simulink library "tqr"  (R2021b)
settings: Solver=VariableStepAuto  StartTime=0.0  StopTime=10.0  RelTol=1e-3
undefined symbols (not defined in the file): ATQR_AltRDCActiveFEDUInc_X_pct, ATQR_AltRDCActiveFEDUInc_Y_enum, ATQR_AltRDCActiveFEDUTs_X_pct, ATQR_AltRDCActiveFEDUTs_Y_enum, ATQR_AltRDCActiveREDUInc_X_pct, ATQR_AltRDCActiveREDUInc_Y_enum, ATQR_AltRDCActiveREDUTs_X_pct, ATQR_AltRDCActiveREDUTs_Y_enum, ATQR_CreepFEDUTqIncSR_X_rpm, ATQR_CreepFEDUTqIncSR_Y_Nm, ATQR_CreepFEDUTs_X_rpm, ATQR_CreepFEDUTs_Y_Nm, ATQR_ECO2TqFrIncGain_X_Nm, ATQR_ECO2TqFrIncGain_Y_pct, ATQR_ECO2TqRrIncGain_X_Nm, ATQR_ECO2TqRrIncGain_Y_pct, ATQR_EcoTqFrIncGain_X_Nm, ATQR_EcoTqFrIncGain_Y_pct, ATQR_EcoTqRrIncGain_X_Nm, ATQR_EcoTqRrIncGain_Y_pct, ATQR_EL1FEDUTqDecSR_Y_Nm, ATQR_EL1FEDUTqIncSR_X_rpm, ATQR_EL1FEDUTqIncSR_Y_pct, ATQR_EL1FEDUTs_X_rpm, ATQR_EL1FEDUTs_Y_Nm, ATQR_EL1REDUTqDecSR_Y_Nm, ATQR_EL1REDUTs_Y_Nm, ATQR_FEDUEL1RegenTs_X_rpm, ATQR_FEDUTIPOutTs_X_rpm, ATQR_FrNegRateLimitIncN_X_rpm, ATQR_FrNegRateLimitIncN_Y_Nm, ATQR_FrPosRateLimitIncN_X_rpm, ATQR_FrPosRateLimitIncN_Y_Nm, ATQR_FrPreLoadTqIncSR_X_rpm, ATQR_FrPreLoadTqIncSR_Y_Nm, ATQR_FShaftSpdTqLimCoe_X_rpm, ATQR_FTimerTqLimCoe_X_s, ATQR_FTqZeroTransUpBoundN_X_rpm, ATQR_NL1FEDUTqDecSR_Y_Nm, ATQR_NL1FEDUTqIncSR_X_rpm, ATQR_NL1FEDUTqIncSR_Y_pct, ATQR_NL1FEDUTs_X_rpm, ATQR_NL1FEDUTs_Y_Nm, ATQR_NL1REDUTqDecSR_Y_Nm, ATQR_NL1REDUTs_Y_Nm, ATQR_NL2TqFrIncGain_X_Nm, ATQR_NL2TqFrIncGain_Y_pct, ATQR_NL2TqRrIncGain_X_Nm, ATQR_NL2TqRrIncGain_Y_pct, ATQR_NormalTqFrIncGain_X_Nm, ATQR_NormalTqFrIncGain_Y_pct, ATQR_NormalTqRrIncGain_X_Nm, ATQR_NormalTqRrIncGain_Y_pct, ATQR_RrNegRateLimitIncN_X_rpm, ATQR_RrNegRateLimitIncN_Y_Nm, ATQR_RrPosRateLimitIncN_X_rpm, ATQR_RrPosRateLimitIncN_Y_Nm, ATQR_RrPreLoadTqIncSR_X_rpm, ATQR_RrPreLoadTqIncSR_Y_Nm, ATQR_RShaftSpdTqLimCoe_X_rpm ... (+349)
libraries: hcu_lib x21, simulink x15, $bdroot x3
(part 3 of 12)

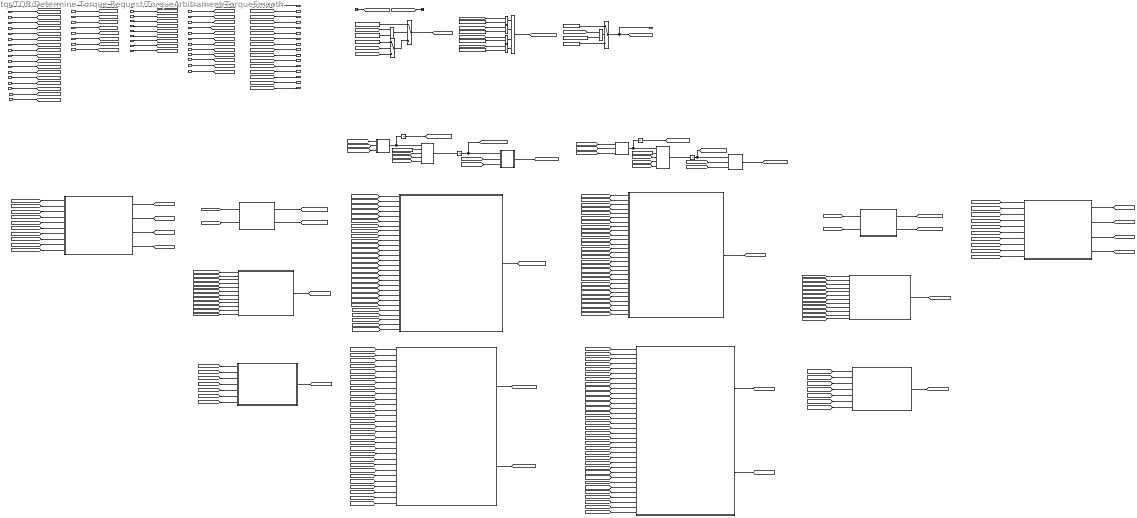
== system tqr/TQR/Determine Torque Request/TorqueArbitrament/TorqueSmooth ==
  note: Fr | Rr
  note: Front First order filter input tau map and determination
  note: Rear Rate limitation map and determination
  note: Front Rate limitation map and determination
  note: Rear wheel first order filter input torque command determination
  note: Front wheel first order filter input torque command determination:
  note: Rear Torque zero point transfer status determination
  note: Front Torque zero point transfer status determination
  note: Front Torque zero point transfer boundary map
  note: Rear Torque zero point transfer boundary map
  note: Rear First order filter input tau map and determination
  note: Rear torque ramp limtation and determination
  note: Rear torque ramp limtation and determination
  note: Rear Final Torque
  note: Front Final Torque
  task_time_s : Inport
  VDHP_ActAPSPosn_pct : Inport  Port=2
  VTQD_TqTargetShaftSpd_rpm : Inport  Port=3
  VTQD_TqSourceFr_enum : Inport  Port=4
  VTQD_TqSourceRr_enum : Inport  Port=5
  VTQD_AfterAvailableTqDemRr_Nm : Inport  Port=6
  VTQD_AfterAvailableTqDemFr_Nm : Inport  Port=7
  VTQD_EVDriveMode_enum : Inport  Port=8
  VTQD_EVDriveModeValid_flg : Inport  Port=9
  VTQD_RollRegenEnable_flg : Inport  Port=10
  VINP_VehSpeed_kph : Inport  Port=11
  VPMM_DriveTrainSelect_enum : Inport  Port=12
  VTQD_LimpHomeAct_flg : Inport  Port=13
  VTQD_RegenMode_enum : Inport  Port=14
  VVMC_ACCPedalOvrd_flg : Inport  Port=15
  VVMC_CCPedalOvrd_flg : Inport  Port=16
  VTQD_GearActualPosn_enum : Inport  Port=17
  VTQD_PreLoadHold_flg : Inport  Port=18
  VTQD_PreLoadPreEn_flg : Inport  Port=19
  VTQR_NoABSFEDUWhlTqReq_Nm : Inport  Port=20
  VTQR_NoABSREDUWhlTqReq_Nm : Inport  Port=21
  VTQD_CreepPrLoadEnable_flg : Inport  Port=22
  VVMC_ADASActive_flg : Inport  Port=23
  VTQD_RDCActive_enum : Inport  Port=24
  VVMC_ActMaxSlideRate_pct : Inport  Port=25
  VTQD_RegenTqLimitEn_flg : Inport  Port=26
  VTQD_PedAccTqEn_flg : Inport  Port=27
  VTQR_FrGearChange_flg : Inport  Port=28
  VTQR_RrGearChange_flg : Inport  Port=29
  VVMC_MSAWhlTqActive_flg : Inport  Port=30
  VINP_LFRawWhlSpeed_kph : Inport  Port=31
  VINP_RFRawWhlSpeed_kph : Inport  Port=32
  VINP_LRRawWhlSpeed_kph : Inport  Port=33
  VINP_RRRawWhlSpeed_kph : Inport  Port=34
  VINP_ACCVehHoldReq_flg : Inport  Port=35
  VTQD_VehActSpd_kph : Inport  Port=36
  VVMC_EstSlope_Deg : Inport  Port=37
  VINP_RrPTCSActive_flg : Inport  Port=38
  VINP_FrPTCSActive_flg : Inport  Port=39
  VINP_IVISnowModeCmd_flg : Inport  Port=40
  VINP_VehicleType_enum : Inport  Port=41
  VTQD_LowIdleAccPedal_flg : Inport  Port=42
  VTQD_FrShaftSpd_rpm : Inport  Port=43
  VTQD_RrShaftSpd_rpm : Inport  Port=44
  VINP_ABSActive_flg : Inport  Port=45
  VTQD_IVIRockModeEn_flg : Inport  Port=46
  VINP_FrntAxlTrqReqDrv_Nm : Inport  Port=47
  VINP_RearAxlTrqReqDrv_Nm : Inport  Port=48
  VTQD_CoordWhlTqDemFr_Nm : Inport  Port=49
  VTQD_CoordWhlTqDemRr_Nm : Inport  Port=50
  AND : Logic  Inputs=4  AllPortsSameDT=off  OutDataTypeStr=boolean
  Constant : Constant  Value=ZERO_FLOAT
  Constant1 : Constant  Value=ZERO_FLOAT
  Constant2 : Constant  Value=ENUM_REGENLEVEL_LV1
  Constant3 : Constant  Value=MINUSONE_FLOAT
  Constant4 : Constant  Value=ENUM_DRIVEMODE_SPORT
  Constant5 : Constant  Value=KTQR_LaunchEnPedal_pct
  Constant6 : Constant  Value=KTQR_LaunchEnSpd_kph
  Constant7 : Constant  Value=ONE_FLOAT
  Equal{,1..3} (4 alike) : RelationalOperator  Operator===  OutDataTypeStr=boolean  RndMeth=Simplest
  FirstOrderFilter : Subsystem  RTWFileName=HCU_LIB  mask(FirstOrderFilter){}
      mask help: First order Filter.
      settings: RTWFileNameOpts=User specified
  FirstOrderFilter1 : $bdroot/TQR/Determine Torque Request/TorqueArbitrament/TorqueSmooth/FirstOrderFilter
  Front First order filter input tau map and determination : Subsystem  AncestorBlock=tqr0/TQR/Determine Torque Request/TorqueArbitrament/TorqueSmooth/Front First order filter input tau map and determination
  Front Torque zero point transfer boundary map : Subsystem
  "Front Torque zero point transfer status determination " : Subsystem
  Front torque ramp limtation and determination : Subsystem  AncestorBlock=tqr0/TQR/Determine Torque Request/TorqueArbitrament/TorqueSmooth/Front torque ramp limtation and determination
  Front wheel first order filter input torque command determination : Subsystem  AncestorBlock=tqr0/TQR/Determine Torque Request/TorqueArbitrament/TorqueSmooth/Front wheel first order filter input torque command determination
  Front wheel rate limit determination : Subsystem  AncestorBlock=tqr0/TQR/Determine Torque Request/TorqueArbitrament/TorqueSmooth/Front wheel rate limit determination
  Ground1 : Ground
  Limit : Subsystem  RTWFileName=HCU_LIB  mask(Limit){}
      mask help: Limit funcion.
      settings: RTWFileNameOpts=User specified
  Limit2 : $bdroot/TQR/Determine Torque Request/TorqueArbitrament/TorqueSmooth/Limit
  RateLimit : Subsystem  RTWFileName=HCU_LIB  mask(RateLimit){}
      mask help: Rate limit function.
      settings: RTWFileNameOpts=User specified
  RateLimit1 : $bdroot/TQR/Determine Torque Request/TorqueArbitrament/TorqueSmooth/RateLimit
  Rear First order filter input tau map and determination : Subsystem  AncestorBlock=tqr0/TQR/Determine Torque Request/TorqueArbitrament/TorqueSmooth/Rear First order filter input tau map and determination
  Rear Torque zero point transfer boundary map : Subsystem
  "Rear Torque zero point transfer status determination " : Subsystem
  Rear torque ramp limtation and determination : Subsystem  AncestorBlock=tqr0/TQR/Determine Torque Request/TorqueArbitrament/TorqueSmooth/Rear torque ramp limtation and determination
  Rear wheel first order filter input torque command determination : Subsystem  AncestorBlock=tqr0/TQR/Determine Torque Request/TorqueArbitrament/TorqueSmooth/Rear wheel first order filter input torque command determination
  Rear wheel rate limit determination1 : Subsystem  AncestorBlock=tqr0/TQR/Determine Torque Request/TorqueArbitrament/TorqueSmooth/Rear wheel rate limit determination
  RegenLV_inc1 : Constant  Value=ENUM_GEARACTUALPOSN_R
  RegenLV_inc2 : Constant  Value=ENUM_DRIVEMODE_ECO
  RegenLV_inc5 : Constant  Value=ENUM_GEARACTUALPOSN_R
  RegenLV_inc6 : Constant  Value=ENUM_DRIVEMODE_NRM
  Relational Operator4 : RelationalOperator  Operator=>  OutDataTypeStr=boolean  RndMeth=Simplest
  Relational Operator6 : RelationalOperator  Operator=<=  OutDataTypeStr=boolean  RndMeth=Simplest
  Switch : Switch  Criteria=u2 ~= 0
  Switch1 : Switch  Criteria=u2 > Threshold
  Switch2 : Switch  Criteria=u2 ~= 0
  Terminator2 : Terminator
  Unit Delay{1..4} (4 alike) : UnitDelay  SampleTime=-1
  VTQR_RampFEDUWhlTqReq_Nm : Outport
  VTQR_RampREDUWhlTqReq_Nm : Outport  Port=2
  VTQR_RampTqCMDGain_c : Outport  Port=3
  VTQR_RShaftSpdTqLimLow_flg : Outport  Port=4
  VTQR_RTimerTqLimLow_flg : Outport  Port=5
  VTQR_FShaftSpdTqLimLow_flg : Outport  Port=6
  VTQR_FTimerTqLimLow_flg : Outport  Port=7
  VTQR_FrFirstOrderInpTs_c : Outport  Port=8
  VTQR_RrFirstOrderInpTs_c : Outport  Port=9
  VTQR_FrRateLimitInc_Nm : Outport  Port=10
  VTQR_FrRateLimitDec_Nm : Outport  Port=11
  VTQR_RrRateLimitInc_Nm : Outport  Port=12
  VTQR_RrRateLimitDec_Nm : Outport  Port=13
  VTQR_FrTqZeroTransLowBound_Nm : Outport  Port=14
  VTQR_RrTqZeroTransUpBound_Nm : Outport  Port=15
  VTQR_FrTqZeroTrans_enum : Outport  Port=16
  VTQR_RrTqZeroTrans_enum : Outport  Port=17
  wires:
  [task_time_s] -> FirstOrderFilter/2(Tc)
  FirstOrderFilter/1(out) -> Unit Delay3/1, RateLimit/1(input_raw)  "VTQR_FrFirstOrderOutTq_Nm"
  task_time_s/1 -> [task_time_s]
  RateLimit/1(output) -> Unit Delay1/1  "VTQR_FEDUWhlTqReqSmooth_Nm"
  Unit Delay1/1 -> [VTQR_FEDUWhlTqReqSmoothDelay_Nm], Limit/1(input)  "VTQR_FEDUWhlTqReqSmoothDelay_Nm"
  [VTQR_ActFEDUTrqUpLim_Nm] -> Limit/2(upper_limit)
  [VTQR_ActFEDUTrqLowLim_Nm] -> Limit/3(lower_limit)
  Limit/1(out) -> [VTQR_RampFEDUWhlTqReq_Nm]  "VTQR_RampFEDUWhlTqReq_Nm"
  [task_time_s] -> RateLimit/3(steptime)
  Constant/1 -> RateLimit/2(initial_value)
  VTQD_TqSourceFr_enum/1 -> [VTQD_TqSourceFr_enum]
  VDHP_ActAPSPosn_pct/1 -> [VDHP_ActAPSPosn_pct]
  VTQD_AfterAvailableTqDemFr_Nm/1 -> [VTQD_AfterAvailableTqDemFr_Nm]
  VTQD_AfterAvailableTqDemRr_Nm/1 -> [VTQD_AfterAvailableTqDemRr_Nm]
  Unit Delay2/1 -> [VTQR_REDUWhlTqReqSmoothDelay_Nm], Limit2/1  "VTQR_REDUWhlTqReqSmoothDelay_Nm"
  RateLimit1/1 -> Unit Delay2/1  "VTQR_REDUWhlTqReqSmooth_Nm"
  FirstOrderFilter1/1 -> Unit Delay4/1, RateLimit1/1  "VTQR_RrFirstOrderOutTq_Nm"
  [task_time_s] -> FirstOrderFilter1/2
  Limit2/1 -> [VTQR_RampREDUWhlTqReq_Nm]  "VTQR_RampREDUWhlTqReq_Nm"
  [task_time_s] -> RateLimit1/3
  Constant1/1 -> RateLimit1/2
  VTQD_EVDriveMode_enum/1 -> [VTQD_EVDriveMode_enum]
  VTQD_RollRegenEnable_flg/1 -> [VTQD_RollRegenEnable_flg]
  VINP_VehSpeed_kph/1 -> [VINP_VehSpeed_kph]
  VPMM_DriveTrainSelect_enum/1 -> [VPMM_DriveTrainSelect_enum]
  VTQD_LimpHomeAct_flg/1 -> [VTQD_LimpHomeAct_flg]
  VTQD_EVDriveModeValid_flg/1 -> [VTQD_EVDriveModeValid_flg]
  VTQD_TqSourceRr_enum/1 -> [VTQD_TqSourceRr_enum]
  Front wheel first order filter input torque command determination/1(VTQR_FrFirstOrderInpTq_Nm) -> [VTQR_FrFirstOrderInpTq_Nm]
  Rear wheel first order filter input torque command determination/1(VTQR_RrFirstOrderInpTq_Nm) -> [VTQR_RrFirstOrderInpTq_Nm]
  Front wheel rate limit determination/2(VTQR_FrRateLimitDec_Nm) -> [VTQR_FrRateLimitDec_Nm]
  Front wheel rate limit determination/1(VTQR_FrRateLimitInc_Nm) -> [VTQR_FrRateLimitInc_Nm]
  [VTQR_FrFirstOrderInpTq_Nm] -> FirstOrderFilter/1(in)
  [VTQR_RrFirstOrderInpTq_Nm] -> FirstOrderFilter1/1
  [VTQR_FrRateLimitInc_Nm] -> RateLimit/4(ratelimt_inc)
  [VTQR_FrRateLimitDec_Nm] -> RateLimit/5(ratelimt_dec)
  Rear wheel rate limit determination1/1(VTQR_RrRateLimitInc_Nm) -> [VTQR_RrRateLimitInc_Nm]
  [VTQR_RrRateLimitInc_Nm] -> RateLimit1/4
  [VTQR_RrRateLimitDec_Nm] -> RateLimit1/5
  Unit Delay3/1 -> [VTQR_FrFirstOrderOutTqDelay_Nm]  "VTQR_FrFirstOrderOutTqDelay_Nm"
  Front First order filter input tau map and determination/1(VTQR_FrFirstOrderInpTs_c) -> [VTQR_FrFirstOrderInpTs_c]
  [VTQR_FrFirstOrderInpTs_c] -> FirstOrderFilter/3(Ts)
  Rear First order filter input tau map and determination/1(VTQR_RrFirstOrderInpTs_c) -> [VTQR_RrFirstOrderInpTs_c]
  [VTQR_RrFirstOrderInpTs_c] -> FirstOrderFilter1/3
  Unit Delay4/1 -> [VTQR_RrFirstOrderOutTqDelay_Nm]  "VTQR_RrFirstOrderOutTqDelay_Nm"
  [VTQD_TqTargetShaftSpd_rpm] -> Front First order filter input tau map and determination/1(VTQD_TqTargetShaftSpd_rpm)
  [VTQR_EVDriveMode_enum] -> Front First order filter input tau map and determination/2(VTQR_EVDriveMode_enum)
  [VTQD_RollRegenEnable_flg] -> Front First order filter input tau map and determination/3(VTQD_RollRegenEnable_flg)
  [VTQD_TqSourceFr_enum] -> Front First order filter input tau map and determination/4(VTQD_TqSourceFr_enum)
  [VTQR_FEDUWhlTqReqSmoothDelay_Nm] -> Front First order filter input tau map and determination/5(VTQR_FEDUWhlTqReqSmoothDelay_Nm)
  [VDHP_ActAPSPosn_pct] -> Front First order filter input tau map and determination/6(VDHP_ActAPSPosn_pct)
  [VINP_VehSpeed_kph] -> Front First order filter input tau map and determination/7(VINP_VehSpeed_kph)
  [VTQD_LimpHomeAct_flg] -> Front First order filter input tau map and determination/8(VTQD_LimpHomeAct_flg)
  [VTQD_TqTargetShaftSpd_rpm] -> Rear First order filter input tau map and determination/1(VTQD_TqTargetShaftSpd_rpm)
  [VTQR_EVDriveMode_enum] -> Rear First order filter input tau map and determination/2(VTQR_EVDriveMode_enum)
  [VTQD_RollRegenEnable_flg] -> Rear First order filter input tau map and determination/3(VTQD_RollRegenEnable_flg)
  [VTQD_TqSourceRr_enum] -> Rear First order filter input tau map and determination/4(VTQD_TqSourceRr_enum)
  [VTQR_REDUWhlTqReqSmoothDelay_Nm] -> Rear First order filter input tau map and determination/5(VTQR_REDUWhlTqReqSmooth_Nm)
  [VDHP_ActAPSPosn_pct] -> Rear First order filter input tau map and determination/6(VDHP_ActAPSPosn_pct)
  [VINP_VehSpeed_kph] -> Rear First order filter input tau map and determination/7(VINP_VehSpeed_kph)
  [VTQD_LimpHomeAct_flg] -> Rear First order filter input tau map and determination/8(VTQD_LimpHomeAct_flg)
  [VTQD_EVDriveModeValid_flg] -> Rear First order filter input tau map and determination/9(VTQD_EVDriveModeValid_flg)
  [VTQD_EVDriveModeValid_flg] -> Front First order filter input tau map and determination/9(VTQD_EVDriveModeValid_flg)
  [VTQD_TqTargetShaftSpd_rpm] -> Front Torque zero point transfer boundary map/1(VTQD_TqTargetShaftSpd_rpm)
  [VTQR_EVDriveMode_enum] -> Front Torque zero point transfer boundary map/2(VTQR_EVDriveMode_enum)
  Front Torque zero point transfer boundary map/1(VTQR_FrTqZeroTransUpBound_Nm) -> [VTQR_FrTqZeroTransUpBound_Nm]
  Front Torque zero point transfer boundary map/2(VTQR_FrTqZeroTransLowBound_Nm) -> [VTQR_FrTqZeroTransLowBound_Nm]
  [VTQD_TqTargetShaftSpd_rpm] -> Rear Torque zero point transfer boundary map/1(VTQD_TqTargetShaftSpd_rpm)
  [VTQR_EVDriveMode_enum] -> Rear Torque zero point transfer boundary map/2(VTQR_EVDriveMode_enum)
  Rear Torque zero point transfer boundary map/1(VTQR_RrTqZeroTransUpBound_Nm) -> [VTQR_RrTqZeroTransUpBound_Nm]
  Rear Torque zero point transfer boundary map/2(VTQR_RrTqZeroTransLowBound_Nm) -> [VTQR_RrTqZeroTransLowBound_Nm]
  [VTQD_RegenMode_enum] -> Front First order filter input tau map and determination/10(VTQD_RegenMode_enum)
  VTQD_RegenMode_enum/1 -> [VTQD_RegenMode_enum]
  [VTQD_RegenMode_enum] -> Rear First order filter input tau map and determination/10(VTQD_RegenMode_enum)
  VVMC_ACCPedalOvrd_flg/1 -> [VVMC_ACCPedalOvrd_flg]
  VVMC_CCPedalOvrd_flg/1 -> [VVMC_CCPedalOvrd_flg]
  RegenLV_inc5/1 -> Equal/2
  Equal/1 -> Switch/2
  RegenLV_inc6/1 -> Switch/1
  Switch/1 -> [VTQR_EVDriveMode_enum]  "VTQR_EVDriveMode_enum"
  [VTQD_GearActualPosn_enum] -> Equal/1
  VTQD_GearActualPosn_enum/1 -> [VTQD_GearActualPosn_enum]
  [VVMC_ACCPedalOvrd_flg] -> Rear First order filter input tau map and determination/11(VVMC_ACCPedalOvrd_flg)
  [VVMC_CCPedalOvrd_flg] -> Rear First order filter input tau map and determination/12(VVMC_CCPedalOvrd_flg)
  VTQD_TqTargetShaftSpd_rpm/1 -> [VTQD_TqTargetShaftSpd_rpm]
  VTQD_PreLoadHold_flg/1 -> [VTQD_PreLoadHold_flg]
  VTQD_PreLoadPreEn_flg/1 -> [VTQD_PreLoadPreEn_flg]
  [VTQD_PreLoadHold_flg] -> Rear First order filter input tau map and determination/13(VTQD_PreLoadHold_flg)
  VTQR_NoABSFEDUWhlTqReq_Nm/1 -> [VTQR_NoABSFEDUWhlTqReq_Nm]
  VTQR_NoABSREDUWhlTqReq_Nm/1 -> [VTQR_NoABSREDUWhlTqReq_Nm]
  VTQD_CreepPrLoadEnable_flg/1 -> [VTQD_CreepPrLoadEnable_flg]
  VVMC_ADASActive_flg/1 -> [VVMC_ADASActive_flg]
  [VTQD_CreepPrLoadEnable_flg] -> Rear First order filter input tau map and determination/15(VTQD_CreepPrLoadEnable_flg)
  VTQD_RDCActive_enum/1 -> [VTQD_RDCActive_enum]
  Ground1/1 -> [VINP_SCPSystemMode_enum]
  [VTQD_RDCActive_enum] -> Rear First order filter input tau map and determination/16(VTQD_RDCActive_enum)
  [VTQR_NoABSREDUWhlTqReq_Nm] -> Rear First order filter input tau map and determination/17(VTQR_NoABSREDUWhlTqReq_Nm)
  [VTQR_RampREDUWhlTqReq_Nm] -> Rear First order filter input tau map and determination/18(VTQR_RampREDUWhlTqReq_Nm)
  [VTQR_RrFirstOrderInpTq_Nm] -> Rear First order filter input tau map and determination/19(VTQR_RrFirstOrderInpTq_Nm)
  [VTQR_ActREDUTrqUpLim_Nm] -> Limit2/2
  [VTQR_ActREDUTrqLowLim_Nm] -> Limit2/3
  VVMC_ActMaxSlideRate_pct/1 -> [VVMC_ActMaxSlideRate_pct]
  VTQD_RegenTqLimitEn_flg/1 -> [VTQD_RegenTqLimitEn_flg]
  VTQD_PedAccTqEn_flg/1 -> [VTQD_PedAccTqEn_flg]
  [VVMC_ActMaxSlideRate_pct] -> Rear First order filter input tau map and determination/14(VVMC_ActMaxSlideRate_pct)
  [VTQD_PedAccTqEn_flg] -> Rear First order filter input tau map and determination/20(VTQD_PedAccTqEn_flg)
  Constant5/1 -> Relational Operator4/2
  Relational Operator4/1 -> AND/1
  Equal2/1 -> AND/4
  [VTQR_EVDriveMode_enum] -> Equal1/1
  Equal1/1 -> AND/3
  [VDHP_ActAPSPosn_pct] -> Relational Operator4/1
  [VINP_VehSpeed_kph] -> Relational Operator6/1
  Relational Operator6/1 -> AND/2
  AND/1 -> [VTQR_LaunchEn_flg]  "VTQR_LaunchEn_flg"
  [VTQD_RegenMode_enum] -> Equal2/1
  Constant6/1 -> Relational Operator6/2
  Constant2/1 -> Equal2/2
  Constant4/1 -> Equal1/2
  [VTQR_RampFEDUWhlTqReq_Nm] -> VTQR_RampFEDUWhlTqReq_Nm/1  "VTQR_RampFEDUWhlTqReq_Nm"
  [VTQR_RampREDUWhlTqReq_Nm] -> VTQR_RampREDUWhlTqReq_Nm/1  "VTQR_RampREDUWhlTqReq_Nm"
  [VTQR_FrGearChange_flg] -> Front wheel first order filter input torque command determination/6(VTQR_FrGearChange_flg)
  [VTQR_FrFirstOrderOutTqDelay_Nm] -> Front wheel first order filter input torque command determination/5(VTQR_FrFirstOrderOutTqDelay_Nm)
  [VTQR_FrTqZeroTrans_enum] -> Front wheel first order filter input torque command determination/1(VTQR_FrTqZeroTrans_enum)
  [VTQD_AfterAvailableTqDemFr_Nm] -> Front wheel first order filter input torque command determination/4(VTQD_AfterAvailableTqDemFr_Nm)
  [VTQR_FrTqZeroTransLowBound_Nm] -> Front wheel first order filter input torque command determination/3(VTQR_FrTqZeroTransLowBound_Nm)
  [VTQR_FrTqZeroTransUpBound_Nm] -> Front wheel first order filter input torque command determination/2(VTQR_FrTqZeroTransUpBound_Nm)
  [VTQR_RrGearChange_flg] -> Rear wheel first order filter input torque command determination/6(VTQR_RrGearChange_flg)
  [VTQR_RrTqZeroTransUpBound_Nm] -> Rear wheel first order filter input torque command determination/2(VTQR_RrTqZeroTransUpBound_Nm)
  [VTQD_AfterAvailableTqDemRr_Nm] -> Rear wheel first order filter input torque command determination/4(VTQD_AfterAvailableTqDemRr_Nm)
  [VTQR_RrTqZeroTransLowBound_Nm] -> Rear wheel first order filter input torque command determination/3(VTQR_RrTqZeroTransLowBound_Nm)
  [VTQR_RrFirstOrderOutTqDelay_Nm] -> Rear wheel first order filter input torque command determination/5(VTQR_RrFirstOrderOutTqDelay_Nm)
  [VTQR_RrTqZeroTrans_enum] -> Rear wheel first order filter input torque command determination/1(VTQR_RrTqZeroTrans_enum)
  VTQR_RrGearChange_flg/1 -> [VTQR_RrGearChange_flg]
  VTQR_FrGearChange_flg/1 -> [VTQR_FrGearChange_flg]
  [VINP_SCPSystemMode_enum] -> Terminator2/1
  [VTQD_PreLoadPreEn_flg] -> Rear First order filter input tau map and determination/21(VTQD_PreLoadPreEn_flg)
  RegenLV_inc1/1 -> Equal3/2
  Equal3/1 -> Switch1/2
  [VTQD_GearActualPosn_enum] -> Equal3/1
  Constant3/1 -> Switch1/1
  Constant7/1 -> Switch1/3
  Switch1/1 -> VTQR_RampTqCMDGain_c/1, [VTQR_RampTqCMDGain_c]  "VTQR_RampTqCMDGain_c"
  [VTQR_RampTqCMDGain_c] -> Front wheel first order filter input torque command determination/7(VTQR_RampTqCMDGain_c)
  [VTQR_RampTqCMDGain_c] -> Rear wheel first order filter input torque command determination/7(VTQR_RampTqCMDGain_c)
  VVMC_MSAWhlTqActive_flg/1 -> [VVMC_MSAWhlTqActive_flg]
  [VVMC_MSAWhlTqActive_flg] -> Rear First order filter input tau map and determination/22(VVMC_MSAWhlTqActive_flg)
  [VTQD_AfterAvailableTqDemFr_Nm] -> Front torque ramp limtation and determination/1(VTQD_AfterAvailableTqDemFr_Nm)
  Front torque ramp limtation and determination/2(VTQR_ActFEDUTrqLowLim_Nm) -> [VTQR_ActFEDUTrqLowLim_Nm]
  [VTQD_AfterAvailableTqDemRr_Nm] -> Front torque ramp limtation and determination/2(VTQD_AfterAvailableTqDemRr_Nm)
  Front torque ramp limtation and determination/1(VTQR_ActFEDUTrqUpLim_Nm) -> [VTQR_ActFEDUTrqUpLim_Nm]
  [task_time_s] -> Rear torque ramp limtation and determination/7(task_time_s)
  [VINP_LRRawWhlSpeed_kph] -> Rear torque ramp limtation and determination/5(VINP_LRRawWhlSpeed_kph)
  [VINP_RRRawWhlSpeed_kph] -> Rear torque ramp limtation and determination/6(VINP_RRRawWhlSpeed_kph)
  [VPMM_DriveTrainSelect_enum] -> Rear torque ramp limtation and determination/4(VPMM_DriveTrainSelect_enum)
  [VTQR_FEDUWhlTqReqSmoothDelay_Nm] -> Rear torque ramp limtation and determination/3(VTQR_FEDUWhlTqReqSmoothDelay_Nm)
  [VTQD_AfterAvailableTqDemFr_Nm] -> Rear torque ramp limtation and determination/1(VTQD_AfterAvailableTqDemFr_Nm)
  Rear torque ramp limtation and determination/2(VTQR_ActREDUTrqLowLim_Nm) -> [VTQR_ActREDUTrqLowLim_Nm]
  [VTQD_AfterAvailableTqDemRr_Nm] -> Rear torque ramp limtation and determination/2(VTQD_AfterAvailableTqDemRr_Nm)
  Rear torque ramp limtation and determination/1(VTQR_ActREDUTrqUpLim_Nm) -> [VTQR_ActREDUTrqUpLim_Nm]
  VINP_LFRawWhlSpeed_kph/1 -> [VINP_LFRawWhlSpeed_kph]
  VINP_LRRawWhlSpeed_kph/1 -> [VINP_LRRawWhlSpeed_kph]
  VINP_RRRawWhlSpeed_kph/1 -> [VINP_RRRawWhlSpeed_kph]
  VINP_RFRawWhlSpeed_kph/1 -> [VINP_RFRawWhlSpeed_kph]
  VINP_ACCVehHoldReq_flg/1 -> [VINP_ACCVehHoldReq_flg]
  VTQD_VehActSpd_kph/1 -> [VTQD_VehActSpd_kph]
  [VTQD_PreLoadPreEn_flg] -> "Rear Torque zero point transfer status determination "/6(VTQD_PreLoadPreEn_flg)
  [VVMC_ACCPedalOvrd_flg] -> "Rear Torque zero point transfer status determination "/8(VVMC_ACCPedalOvrd_flg)
  [VINP_VehSpeed_kph] -> "Rear Torque zero point transfer status determination "/12(VINP_VehSpeed_kph)
  [VVMC_EstSlope_Deg] -> "Rear Torque zero point transfer status determination "/9(VVMC_EstSlope_Deg)
  [VTQR_LaunchEn_flg] -> "Rear Torque zero point transfer status determination "/7(VTQR_LaunchEn_flg)
  "Rear Torque zero point transfer status determination "/1(VTQR_RrTqZeroTrans_enum) -> [VTQR_RrTqZeroTrans_enum]
  [VTQD_CreepPrLoadEnable_flg] -> "Rear Torque zero point transfer status determination "/4(VTQD_CreepPrLoadEnable_flg)
  [VTQR_RrTqZeroTransUpBound_Nm] -> "Rear Torque zero point transfer status determination "/2(VTQR_RrTqZeroTransUpBound_Nm)
  [VTQD_AfterAvailableTqDemRr_Nm] -> "Rear Torque zero point transfer status determination "/11(VTQD_AfterAvailableTqDemRr_Nm)
  [VTQD_RegenMode_enum] -> "Rear Torque zero point transfer status determination "/10(VTQD_RegenMode_enum)
  [VTQR_RrTqZeroTransLowBound_Nm] -> "Rear Torque zero point transfer status determination "/3(VTQR_RrTqZeroTransLowBound_Nm)
  [VTQR_REDUWhlTqReqSmoothDelay_Nm] -> "Rear Torque zero point transfer status determination "/1(VTQR_REDUWhlTqReqSmoothDelay_Nm)
  [VVMC_ADASActive_flg] -> "Rear Torque zero point transfer status determination "/5(VVMC_ADASActive_flg)
  VVMC_EstSlope_Deg/1 -> [VVMC_EstSlope_Deg]
  [VTQD_CreepPrLoadEnable_flg] -> "Front Torque zero point transfer status determination "/4(VTQD_CreepPrLoadEnable_flg)
  [VTQR_FrTqZeroTransLowBound_Nm] -> "Front Torque zero point transfer status determination "/3(VTQR_FrTqZeroTransLowBound_Nm)
  [VTQD_PreLoadPreEn_flg] -> "Front Torque zero point transfer status determination "/6(VTQD_PreLoadPreEn_flg)
  [VTQR_LaunchEn_flg] -> "Front Torque zero point transfer status determination "/7(VTQR_LaunchEn_flg)
  [VVMC_EstSlope_Deg] -> "Front Torque zero point transfer status determination "/9(VVMC_EstSlope_Deg)
  [VTQD_AfterAvailableTqDemFr_Nm] -> "Front Torque zero point transfer status determination "/11(VTQD_AfterAvailableTqDemFr_Nm)
  "Front Torque zero point transfer status determination "/1(VTQR_FrTqZeroTrans_enum) -> [VTQR_FrTqZeroTrans_enum]
  [VTQR_FrTqZeroTransUpBound_Nm] -> "Front Torque zero point transfer status determination "/2(VTQR_FrTqZeroTransUpBound_Nm)
  [VVMC_ADASActive_flg] -> "Front Torque zero point transfer status determination "/5(VVMC_ADASActive_flg)
  [VVMC_ACCPedalOvrd_flg] -> "Front Torque zero point transfer status determination "/8(VVMC_ACCPedalOvrd_flg)
  [VTQD_RegenMode_enum] -> "Front Torque zero point transfer status determination "/10(VTQD_RegenMode_enum)
  [VINP_VehSpeed_kph] -> "Front Torque zero point transfer status determination "/12(VINP_VehSpeed_kph)
  [VTQR_FEDUWhlTqReqSmoothDelay_Nm] -> "Front Torque zero point transfer status determination "/1(VTQR_FEDUWhlTqReqSmoothDelay_Nm)
  [VINP_RrPTCSActive_flg] -> Rear First order filter input tau map and determination/23(VINP_RrPTCSActive_flg)
  [VINP_IVISnowModeCmd_flg] -> Rear First order filter input tau map and determination/24(VINP_IVISnowModeCmd_flg)
  VINP_FrPTCSActive_flg/1 -> [VINP_FrPTCSActive_flg]
  VINP_RrPTCSActive_flg/1 -> [VINP_RrPTCSActive_flg]
  VINP_IVISnowModeCmd_flg/1 -> [VINP_IVISnowModeCmd_flg]
  [VINP_IVISnowModeCmd_flg] -> Front First order filter input tau map and determination/24(VINP_IVISnowModeCmd_flg)
  [VTQD_EVDriveMode_enum] -> Switch2/3
  [VINP_IVISnowModeCmd_flg] -> Switch2/2
  RegenLV_inc2/1 -> Switch2/1
  Switch2/1 -> Switch/3
  VINP_VehicleType_enum/1 -> [VINP_VehicleType_enum]
  [VTQR_REDUWhlTqReqSmoothDelay_Nm] -> Front torque ramp limtation and determination/3(VTQR_REDUWhlTqReqSmoothDelay_Nm)
  [VPMM_DriveTrainSelect_enum] -> Front torque ramp limtation and determination/4(VPMM_DriveTrainSelect_enum)
  [VINP_LFRawWhlSpeed_kph] -> Front torque ramp limtation and determination/5(VINP_LFRawWhlSpeed_kph)
  [VINP_RFRawWhlSpeed_kph] -> Front torque ramp limtation and determination/6(VINP_RFRawWhlSpeed_kph)
  [task_time_s] -> Front torque ramp limtation and determination/7(task_time_s)
  VTQD_RrShaftSpd_rpm/1 -> [VTQD_RrShaftSpd_rpm]
  VTQD_FrShaftSpd_rpm/1 -> [VTQD_FrShaftSpd_rpm]
  VTQD_LowIdleAccPedal_flg/1 -> [VTQD_LowIdleAccPedal_flg]
  VINP_ABSActive_flg/1 -> [VINP_ABSActive_flg]
  VTQD_IVIRockModeEn_flg/1 -> [VTQD_IVIRockModeEn_flg]
  [VINP_ABSActive_flg] -> Front torque ramp limtation and determination/8(VINP_ABSActive_flg)
  [VINP_FrPTCSActive_flg] -> Front torque ramp limtation and determination/9(VINP_FrPTCSActive_flg)
  [VTQD_LowIdleAccPedal_flg] -> Front torque ramp limtation and determination/10(VTQD_LowIdleAccPedal_flg)
  Front torque ramp limtation and determination/3(VTQR_FShaftSpdTqLimLow_flg) -> [VTQR_FShaftSpdTqLimLow_flg]
  Front torque ramp limtation and determination/4(VTQR_FTimerTqLimLow_flg) -> [VTQR_FTimerTqLimLow_flg]
  [VTQR_RTimerTqLimLow_flg] -> VTQR_RTimerTqLimLow_flg/1
  [VTQR_FTimerTqLimLow_flg] -> VTQR_FTimerTqLimLow_flg/1
  [VTQR_FShaftSpdTqLimLow_flg] -> VTQR_FShaftSpdTqLimLow_flg/1
  [VTQR_RShaftSpdTqLimLow_flg] -> VTQR_RShaftSpdTqLimLow_flg/1
  [VVMC_ACCPedalOvrd_flg] -> Front First order filter input tau map and determination/11(VVMC_ACCPedalOvrd_flg)
  [VVMC_CCPedalOvrd_flg] -> Front First order filter input tau map and determination/12(VVMC_CCPedalOvrd_flg)
  [VTQD_PreLoadHold_flg] -> Front First order filter input tau map and determination/13(VTQD_PreLoadHold_flg)
  [VVMC_ActMaxSlideRate_pct] -> Front First order filter input tau map and determination/14(VVMC_ActMaxSlideRate_pct)
  [VTQD_CreepPrLoadEnable_flg] -> Front First order filter input tau map and determination/15(VTQD_CreepPrLoadEnable_flg)
  [VTQD_RDCActive_enum] -> Front First order filter input tau map and determination/16(VTQD_RDCActive_enum)
  [VTQR_NoABSFEDUWhlTqReq_Nm] -> Front First order filter input tau map and determination/17(VTQR_NoABSFEDUWhlTqReq_Nm)
  [VTQR_RampFEDUWhlTqReq_Nm] -> Front First order filter input tau map and determination/18(VTQR_RampFEDUWhlTqReq_Nm)
  [VTQR_FrFirstOrderInpTq_Nm] -> Front First order filter input tau map and determination/19(VTQR_FrFirstOrderInpTq_Nm)
  [VTQD_PedAccTqEn_flg] -> Front First order filter input tau map and determination/20(VTQD_PedAccTqEn_flg)
  [VTQD_PreLoadPreEn_flg] -> Front First order filter input tau map and determination/21(VTQD_PreLoadPreEn_flg)
  [VVMC_MSAWhlTqActive_flg] -> Front First order filter input tau map and determination/22(VVMC_MSAWhlTqActive_flg)
  [VINP_FrPTCSActive_flg] -> Front First order filter input tau map and determination/23(VINP_FrPTCSActive_flg)
  [VINP_VehicleType_enum] -> Front First order filter input tau map and determination/26(VINP_VehicleType_enum)
  [VTQD_IVIRockModeEn_flg] -> Front First order filter input tau map and determination/25(VTQD_IVIRockModeEn_flg)
  [VTQR_FrTqZeroTrans_enum] -> Front wheel rate limit determination/1(VTQR_FrTqZeroTrans_enum)
  [VTQD_TqSourceFr_enum] -> Front wheel rate limit determination/2(VTQD_TqSourceFr_enum)
  [VTQD_TqTargetShaftSpd_rpm] -> Front wheel rate limit determination/3(VTQD_TqTargetShaftSpd_rpm)
  [VTQD_LimpHomeAct_flg] -> Front wheel rate limit determination/4(VTQD_LimpHomeAct_flg)
  [VTQR_EVDriveMode_enum] -> Front wheel rate limit determination/5(VTQR_EVDriveMode_enum)
  [VDHP_ActAPSPosn_pct] -> Front wheel rate limit determination/6(VDHP_ActAPSPosn_pct)
  [VTQR_FEDUWhlTqReqSmoothDelay_Nm] -> Front wheel rate limit determination/7(VTQR_FEDUWhlTqReqSmoothDelay_Nm)
  [VTQD_EVDriveModeValid_flg] -> Front wheel rate limit determination/8(VTQD_EVDriveModeValid_flg)
  [VTQD_RegenMode_enum] -> Front wheel rate limit determination/9(VTQD_RegenMode_enum)
  [VVMC_ACCPedalOvrd_flg] -> Front wheel rate limit determination/10(VVMC_ACCPedalOvrd_flg)
  [VVMC_CCPedalOvrd_flg] -> Front wheel rate limit determination/11(VVMC_CCPedalOvrd_flg)
  [VTQD_CreepPrLoadEnable_flg] -> Front wheel rate limit determination/12(VTQD_CreepPrLoadEnable_flg)
  [VTQD_RegenTqLimitEn_flg] -> Front wheel rate limit determination/13(VTQD_RegenTqLimitEn_flg)
  [VTQD_RDCActive_enum] -> Front wheel rate limit determination/14(VTQD_RDCActive_enum)
  [VTQD_PreLoadPreEn_flg] -> Front wheel rate limit determination/15(VTQD_PreLoadPreEn_flg)
  [VTQR_NoABSFEDUWhlTqReq_Nm] -> Front wheel rate limit determination/16(VTQR_NoABSFEDUWhlTqReq_Nm)
  [VTQR_RampFEDUWhlTqReq_Nm] -> Front wheel rate limit determination/17(VTQR_RampFEDUWhlTqReq_Nm)
  [VTQR_FrFirstOrderInpTq_Nm] -> Front wheel rate limit determination/18(VTQR_FrFirstOrderInpTq_Nm)
  [VVMC_ActMaxSlideRate_pct] -> Front wheel rate limit determination/19(VVMC_ActMaxSlideRate_pct)
  [VTQD_PedAccTqEn_flg] -> Front wheel rate limit determination/20(VTQD_PedAccTqEn_flg)
  [VVMC_MSAWhlTqActive_flg] -> Front wheel rate limit determination/21(VVMC_MSAWhlTqActive_flg)
  [VINP_FrPTCSActive_flg] -> Front wheel rate limit determination/22(VINP_FrPTCSActive_flg)
  [VINP_IVISnowModeCmd_flg] -> Front wheel rate limit determination/24(VINP_IVISnowModeCmd_flg)
  [VINP_VehicleType_enum] -> Front wheel rate limit determination/27(VINP_VehicleType_enum)
  [VTQD_GearActualPosn_enum] -> Front wheel rate limit determination/23(VTQD_GearActualPosn_enum)
  [VTQD_IVIRockModeEn_flg] -> Front wheel rate limit determination/25(VTQD_IVIRockModeEn_flg)
  [VTQD_FrShaftSpd_rpm] -> Front wheel rate limit determination/26(VTQD_FrShaftSpd_rpm)
  [VINP_VehicleType_enum] -> Rear First order filter input tau map and determination/26(VINP_VehicleType_enum)
  [VTQD_IVIRockModeEn_flg] -> Rear First order filter input tau map and determination/25(VTQD_IVIRockModeEn_flg)
  [VTQR_RrTqZeroTrans_enum] -> Rear wheel rate limit determination1/1(VTQR_RrTqZeroTrans_enum)
  [VTQD_TqSourceRr_enum] -> Rear wheel rate limit determination1/2(VTQD_TqSourceRr_enum)
  [VTQD_TqTargetShaftSpd_rpm] -> Rear wheel rate limit determination1/3(VTQD_TqTargetShaftSpd_rpm)
  [VTQD_LimpHomeAct_flg] -> Rear wheel rate limit determination1/4(VTQD_LimpHomeAct_flg)
  [VTQR_EVDriveMode_enum] -> Rear wheel rate limit determination1/5(VTQR_EVDriveMode_enum)
  [VDHP_ActAPSPosn_pct] -> Rear wheel rate limit determination1/6(VDHP_ActAPSPosn_pct)
  [VTQR_REDUWhlTqReqSmoothDelay_Nm] -> Rear wheel rate limit determination1/7(VTQR_REDUWhlTqReqSmoothDelay_Nm)
  [VTQD_EVDriveModeValid_flg] -> Rear wheel rate limit determination1/8(VTQD_EVDriveModeValid_flg)
  [VTQD_RegenMode_enum] -> Rear wheel rate limit determination1/9(VTQD_RegenMode_enum)
  [VVMC_ACCPedalOvrd_flg] -> Rear wheel rate limit determination1/10(VVMC_ACCPedalOvrd_flg)
  [VVMC_CCPedalOvrd_flg] -> Rear wheel rate limit determination1/11(VVMC_CCPedalOvrd_flg)
  [VTQD_CreepPrLoadEnable_flg] -> Rear wheel rate limit determination1/12(VTQD_CreepPrLoadEnable_flg)
  [VTQD_RegenTqLimitEn_flg] -> Rear wheel rate limit determination1/13(VTQD_RegenTqLimitEn_flg)
  [VTQD_RDCActive_enum] -> Rear wheel rate limit determination1/14(VTQD_RDCActive_enum)
  [VTQD_PreLoadPreEn_flg] -> Rear wheel rate limit determination1/15(VTQD_PreLoadPreEn_flg)
  [VTQR_NoABSREDUWhlTqReq_Nm] -> Rear wheel rate limit determination1/16(VTQR_NoABSREDUWhlTqReq_Nm)
  [VTQR_RampREDUWhlTqReq_Nm] -> Rear wheel rate limit determination1/17(VTQR_RampREDUWhlTqReq_Nm)
  [VTQR_RrFirstOrderInpTq_Nm] -> Rear wheel rate limit determination1/18(VTQR_RrFirstOrderInpTq_Nm)
  [VVMC_ActMaxSlideRate_pct] -> Rear wheel rate limit determination1/19(VVMC_ActMaxSlideRate_pct)
  [VTQD_PedAccTqEn_flg] -> Rear wheel rate limit determination1/20(VTQD_PedAccTqEn_flg)
  [VVMC_MSAWhlTqActive_flg] -> Rear wheel rate limit determination1/21(VVMC_MSAWhlTqActive_flg)
  [VINP_RrPTCSActive_flg] -> Rear wheel rate limit determination1/22(VINP_RrPTCSActive_flg)
  [VINP_IVISnowModeCmd_flg] -> Rear wheel rate limit determination1/24(VINP_IVISnowModeCmd_flg)
  [VVMC_EstSlope_Deg] -> Rear wheel rate limit determination1/27(VVMC_EstSlope_Deg)
  [VTQD_VehActSpd_kph] -> Rear wheel rate limit determination1/28(VTQD_VehActSpd_kph)
  [VVMC_ADASActive_flg] -> Rear wheel rate limit determination1/31(VVMC_ADASActive_flg)
  [VINP_VehicleType_enum] -> Rear wheel rate limit determination1/32(VINP_VehicleType_enum)
  [VPMM_DriveTrainSelect_enum] -> Rear wheel rate limit determination1/30(VPMM_DriveTrainSelect_enum)
  [VINP_ACCVehHoldReq_flg] -> Rear wheel rate limit determination1/29(VINP_ACCVehHoldReq_flg)
  Rear wheel rate limit determination1/2(VTQR_RrRateLimitDec_Nm) -> [VTQR_RrRateLimitDec_Nm]
  [VTQD_GearActualPosn_enum] -> Rear wheel rate limit determination1/23(VTQD_GearActualPosn_enum)
  [VTQD_IVIRockModeEn_flg] -> Rear wheel rate limit determination1/25(VTQD_IVIRockModeEn_flg)
  [VTQD_RrShaftSpd_rpm] -> Rear wheel rate limit determination1/26(VTQD_RrShaftSpd_rpm)
  [VINP_RrPTCSActive_flg] -> Rear torque ramp limtation and determination/8(VINP_RrPTCSActive_flg)
  [VINP_ABSActive_flg] -> Rear torque ramp limtation and determination/9(VINP_ABSActive_flg)
  [VTQD_LowIdleAccPedal_flg] -> Rear torque ramp limtation and determination/10(VTQD_LowIdleAccPedal_flg)
  Rear torque ramp limtation and determination/3(VTQR_RShaftSpdTqLimLow_flg) -> [VTQR_RShaftSpdTqLimLow_flg]
  Rear torque ramp limtation and determination/4(VTQR_RTimerTqLimLow_flg) -> [VTQR_RTimerTqLimLow_flg]
  VTQD_CoordWhlTqDemRr_Nm/1 -> [VTQD_CoordWhlTqDemRr_Nm]
  VTQD_CoordWhlTqDemFr_Nm/1 -> [VTQD_CoordWhlTqDemFr_Nm]
  VINP_RearAxlTrqReqDrv_Nm/1 -> [VINP_RearAxlTrqReqDrv_Nm]
  VINP_FrntAxlTrqReqDrv_Nm/1 -> [VINP_FrntAxlTrqReqDrv_Nm]
  [VTQD_CoordWhlTqDemFr_Nm] -> Front First order filter input tau map and determination/27(VTQD_CoordWhlTqDemFr_Nm)
  [VINP_FrntAxlTrqReqDrv_Nm] -> Front First order filter input tau map and determination/28(VINP_FrntAxlTrqReqDrv_Nm)
  [VTQD_CoordWhlTqDemFr_Nm] -> Front wheel rate limit determination/28(VTQD_CoordWhlTqDemFr_Nm)
  [VINP_FrntAxlTrqReqDrv_Nm] -> Front wheel rate limit determination/29(VINP_FrntAxlTrqReqDrv_Nm)
  [VTQD_CoordWhlTqDemRr_Nm] -> Rear First order filter input tau map and determination/27(VTQD_CoordWhlTqDemRr_Nm)
  [VINP_RearAxlTrqReqDrv_Nm] -> Rear First order filter input tau map and determination/28(VINP_RearAxlTrqReqDrv_Nm)
  [VTQD_CoordWhlTqDemRr_Nm] -> Rear wheel rate limit determination1/33(VTQD_CoordWhlTqDemRr_Nm)
  [VINP_RearAxlTrqReqDrv_Nm] -> Rear wheel rate limit determination1/34(VINP_RearAxlTrqReqDrv_Nm)
  [VTQR_FrFirstOrderInpTs_c] -> VTQR_FrFirstOrderInpTs_c/1
  [VTQR_FrRateLimitDec_Nm] -> VTQR_FrRateLimitDec_Nm/1
  [VTQR_RrRateLimitDec_Nm] -> VTQR_RrRateLimitDec_Nm/1
  [VTQR_RrRateLimitInc_Nm] -> VTQR_RrRateLimitInc_Nm/1
  [VTQR_FrRateLimitInc_Nm] -> VTQR_FrRateLimitInc_Nm/1
  [VTQR_RrFirstOrderInpTs_c] -> VTQR_RrFirstOrderInpTs_c/1
  [VTQR_FrTqZeroTransLowBound_Nm] -> VTQR_FrTqZeroTransLowBound_Nm/1
  [VTQR_RrTqZeroTransUpBound_Nm] -> VTQR_RrTqZeroTransUpBound_Nm/1
  [VTQR_FrTqZeroTrans_enum] -> VTQR_FrTqZeroTrans_enum/1
  [VTQR_RrTqZeroTrans_enum] -> VTQR_RrTqZeroTrans_enum/1

== system tqr/TQR/Determine Torque Request/TorqueArbitrament/TorqueSmooth/FirstOrderFilter ==
  in : Inport
  Tc : Inport  Port=2
  Ts : Inport  Port=3
  Add : Sum
  Add2 : Sum  Inputs=+-
  Constant3 : Constant  OutDataTypeStr=single
  Constant4 : Constant  Value=0  OutDataTypeStr=single
  Constant5 : Constant  Value=0  OutDataTypeStr=single
  Constant6 : Constant  Value=eps  OutDataTypeStr=single
  Divide : Product  Inputs=*/
  MinMax{1..4} (4 alike) : MinMax  Function=max  Inputs=2
  Product : Product  RndMeth=Zero
  Product1 : Product  RndMeth=Zero
  Unit Delay : UnitDelay  SampleTime=-1  HasFrameUpgradeWarning=on
  out : Outport
  wires:
  Add/1 -> out/1, Unit Delay/1
  Divide/1 -> Product1/1, Add2/2
  Constant3/1 -> Add2/1
  Add2/1 -> Product/2
  Product/1 -> Add/1
  Unit Delay/1 -> Product/1
  in/1 -> Product1/2
  Product1/1 -> Add/2
  Tc/1 -> MinMax2/1
  Constant4/1 -> MinMax2/2
  Ts/1 -> MinMax3/1
  Constant5/1 -> MinMax3/2
  MinMax3/1 -> MinMax1/2
  MinMax2/1 -> Divide/1, MinMax1/1
  MinMax1/1 -> MinMax4/1
  Constant6/1 -> MinMax4/2
  MinMax4/1 -> Divide/2
